simulink model "n99tot96reg55neu_10_8p"  (R2022b)
settings: Solver=VariableStepAuto  StartTime=0.0  StopTime=10.0  RelTol=1e-3
libraries: neural x61
(part 3 of 3)

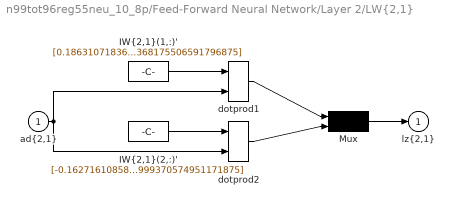
== system n99tot96reg55neu_10_8p/Feed-Forward Neural Network/Layer 2/LW{2,1} ==
  "ad{2,1}" : Inport  PortDimensions=55
      mask Display: e = 0.06;c1 = [120 230 180]/255;c2 = ([120 230 180]+0)/(256+128);c3 = ([120 230 180]+128)/(256+128);patch([0 1 1 0],[0 0 1 1],c1);patch([0 1 1 1-e 1-e 0+e],[0 0 1 1-e 0+e 0+e],c2);patch([0 0 1 1-e 0+e 0+e],[0 1 1 1-e 1-e 0+e],c3);plot([0 1 1 0 0],[0 0 1 1 0]);
  "IW{2,1}(1,:)'" : Constant  Value=[0.1863107183665277666317905413961852900683879852294921875;-1.1925303173738701634221115455147810280323028564453125;0.60630050980529670567875655251555144786834716796875;-0.61044298258553253422320494792074896395206451416015625;0.04135535489732621028391434947479865513741970062255859375;1.487726433617426291533547555445693433284759521484375;1.226968367115052416238540899939835071563720703125;-0.3018571907749816318755620159208774566650390625;5.202381776953959757747725234366953372955322265625;-0.27640862304093338774890753484214656054973602294921875;-0.185523734640249349236995612955070100724697113037109375;-0.2818394795885807990742932815919630229473114013671875;-0.1803306497370077143838074107407010160386562347412109375;0.82910405031643730211499132565222680568695068359375;-1.221384089396997385534859859035350382328033447265625;-0.86513460140942088916204966153600253164768218994140625;0.256827281860183498363170429001911543309688568115234375;-0.5996353591997605203545163021772168576717376708984375;-0.436400005164215343267386515435646288096904754638671875;0.82979567469419723835244440124370157718658447265625;0.70929923288458096575226363711408339440822601318359375;1.172245346408951949257470914744772017002105712890625;-0.0292221833246739427780713782567545422352850437164306640625;-1.2669169119627736730393507968983612954616546630859375;1.53662660536556128221263861632905900478363037109375;-1.13402520630039216342765939771197736263275146484375;1.321388504175650790983809201861731708049774169921875;1.572524953364482058759676874615252017974853515625;-1.005940577470918473323990838252939283847808837890625;1.1644162629613277193385556529392488300800323486328125;0.57547965350007412865807054913602769374847412109375;-1.790392347708127385175203016842715442180633544921875;0.2264605853890448994292228235281072556972503662109375;-1.3676428334882546611339648734428919851779937744140625;-1.0533340168221665411607546047889627516269683837890625;1.1457119697782627287807599714142270386219024658203125;-1.2877378455664632017629855909035541117191314697265625;-0.685795475054770786726976439240388572216033935546875;1.979727820542370064771375837153755128383636474609375;-0.4731114778955320954167973468429408967494964599609375;1.161722316711884417372857569716870784759521484375;1.1136800943773408345549569276045076549053192138671875;-1.331946259277454913672045222483575344085693359375;-1.124914976024559809530956044909544289112091064453125;-1.2982513145884870819912748629576526582241058349609375;-2.11255364859323346848896107985638082027435302734375;-1.4381033364542918917550196056254208087921142578125;-0.79238214971088127835940895238309167325496673583984375;-3.03656782488933263408625862211920320987701416015625;-0.97682792682083474655740928938030265271663665771484375;-0.549880990641058442491839741705916821956634521484375;-0.8056932435256978219939583141240291297435760498046875;0.532594500576840435002168305800296366214752197265625;2.023066814197837626210230155265890061855316162109375;-0.5048197545203823022319511437672190368175506591796875]
      mask Display: e = 0.06;c1 = [120 150 230]/255;c2 = ([120 150 230]+0)/383;c3 = ([120 150 230]+128)/383;patch([0 1 1 0],[0 0 1 1],c1);patch([0 1 1 1-e 1-e 0+e],[0 0 1 1-e 0+e 0+e],c2);patch([0 0 1 1-e 0+e 0+e],[0 1 1 1-e 1-e 0+e],c3);plot([0 1 1 0 0],[0 0 1 1 0]);disp('weights');
  "IW{2,1}(2,:)'" : Constant  Value=[-0.162716108584907537260022536429460160434246063232421875;0.412631133712298148186192747743916697800159454345703125;0.1317397483938761715283050079960958100855350494384765625;-0.1880042522780710212426669158958247862756252288818359375;0.1367064003908134706133381541803828440606594085693359375;-0.94381201649917467744188570577534846961498260498046875;0.404602645293311413698944534189649857580661773681640625;0.390548467497176809981596079524024389684200286865234375;-1.1468896266806860584352989462786354124546051025390625;0.035472913460732273527309388327921624295413494110107421875;-0.1276006599951734210574016969985677860677242279052734375;-0.41033646284198888043448505413834936916828155517578125;0.355232775541665268814739420122350566089153289794921875;0.1874529752752913669411327646230347454547882080078125;0.1516071797516581332043728025382733903825283050537109375;0.1287962746232849953198495995820849202573299407958984375;-1.05750829547899716231995626003481447696685791015625;0.10626001461354088462041289631088147871196269989013671875;0.141864011226467356951985721025266684591770172119140625;-1.3668925384579628801162698437110520899295806884765625;-0.046533509060428433767864220271803787909448146820068359375;0.11202871586376961232645044219680130481719970703125;0.426279212301646170946156644276925362646579742431640625;0.64370945144459046360907450434751808643341064453125;-0.96258471697451108983756284942501224577426910400390625;-0.04251873302794507980539862046498456038534641265869140625;-0.481345772410470773561286250696866773068904876708984375;-0.441823337762237977610624284352525137364864349365234375;-0.56859141224307829798334523729863576591014862060546875;0.0690179888113810202643350066864513792097568511962890625;-0.047488145330204754868130834211115143261849880218505859375;0.37978147788301896969898052702774293720722198486328125;0.260343061208363979464053272749879397451877593994140625;0.09495061983058390719936170398796093650162220001220703125;0.170329364545297623489972238530754111707210540771484375;0.62815733897475289904122064399416558444499969482421875;-0.78674969154341878319058878332725726068019866943359375;-0.08555971922602585710837530541539308615028858184814453125;-0.936562658492846811242316107382066547870635986328125;-0.8804177703487983119856608027475886046886444091796875;-0.052898520213249512755826486909427330829203128814697265625;0.043647654935120218377964107503430568613111972808837890625;0.1322917467071904329412035394852864556014537811279296875;-0.17756019451958493515775217019836418330669403076171875;0.02182726245450583579810199807980097830295562744140625;0.774763537556832915242921444587409496307373046875;0.55134858287374399754554588071187026798725128173828125;-0.168487462360891460111389505982515402138233184814453125;0.64829778292853867949219193178578279912471771240234375;0.2070392982987419860929634296553558669984340667724609375;-0.12395021927616321766318918662364012561738491058349609375;-0.2145476573917964591142748531638062559068202972412109375;-0.8383934255128624446484764121123589575290679931640625;-0.3659025879548252202511093855719082057476043701171875;-0.6102369578631552382574909643153659999370574951171875]
      mask Display: e = 0.06;c1 = [120 150 230]/255;c2 = ([120 150 230]+0)/383;c3 = ([120 150 230]+128)/383;patch([0 1 1 0],[0 0 1 1],c1);patch([0 1 1 1-e 1-e 0+e],[0 0 1 1-e 0+e 0+e],c2);patch([0 0 1 1-e 0+e 0+e],[0 1 1 1-e 1-e 0+e],c3);plot([0 1 1 0 0],[0 0 1 1 0]);disp('weights');
  Mux : Mux  Inputs=2
      mask Display: e = 0.06;c1 = [120 150 230]/255;c2 = ([120 150 230]+0)/383;c3 = ([120 150 230]+128)/383;patch([0 1 1 0],[0 0 1 1],c1);patch([0 1 1 1-e 1-e 0+e],[0 0 1 1-e 0+e 0+e],c2);patch([0 0 1 1-e 0+e 0+e],[0 1 1 1-e 1-e 0+e],c3);plot([0 1 1 0 0],[0 0 1 1 0]);disp('Mux');
  dotprod1 : neural/Weight Functions/dotprod
  dotprod2 : neural/Weight Functions/dotprod
  "lz{2,1}" : Outport
      mask Display: e = 0.06;c1 = [120 230 180]/255;c2 = ([120 230 180]+0)/(256+128);c3 = ([120 230 180]+128)/(256+128);patch([0 1 1 0],[0 0 1 1],c1);patch([0 1 1 1-e 1-e 0+e],[0 0 1 1-e 0+e 0+e],c2);patch([0 0 1 1-e 0+e 0+e],[0 1 1 1-e 1-e 0+e],c3);plot([0 1 1 0 0],[0 0 1 1 0]);
  wires:
  "IW{2,1}(1,:)'"/1 -> dotprod1/1
  "ad{2,1}"/1 -> dotprod1/2, dotprod2/2
  dotprod1/1 -> Mux/1
  "IW{2,1}(2,:)'"/1 -> dotprod2/1
  dotprod2/1 -> Mux/2
  Mux/1 -> "lz{2,1}"/1
